simulink model "tanks"  (R2021b)
settings: Solver=ode45  StartTime=0.0  StopTime=200  RelTol=1e-6  EnableMultiTasking=on
values from neighbouring files (symbols this model uses):
  A_discretized = ssd.A    [control_design.m]
  B_discretized = ssd.B    [control_design.m]
  C = [0 , 1]    [control_design.m]
  C_discretized = ssd.C    [control_design.m]
  D_discretized = ssd.D    [control_design.m]
  F = tf(num, den)    [control_design.m]
  Gamma = sys_d.B    [control_design.m]
  K = acker(transpose(Phi), transpose(C), poles_desiredK).'    [control_design.m]
  L = acker(Phi, Gamma, poles_desiredL)    [control_design.m]
  lr = 1 / (C * inv(I - Phi + Gamma * L) * Gamma)    [control_design.m]
  Phi = sys_d.A    [control_design.m]
  Ts = 4    [control_design.m]
  uss = alpha2/beta*sqrt(2*g*tank_init_h2)*100/15    [control_design.m]
  yss = 40    [control_design.m]
undefined symbols (not defined in the file or in its folder): tank_A1, tank_a1, tank_A2, tank_a2, tank_H1, tank_H2, tank_init_h1, tank_init_h2, tank_Kpump
settings Model: Creator=lindhe  LastModifiedBy=1412
settings SolverCC: AlgebraicLoopSolver=TrustRegion
settings DataIOCC: LimitDataPoints=on  SaveFormat=Array  SignalLoggingSaveFormat=ModelDataLogs  ReturnWorkspaceOutputs=off  SignalLoggingName=sigsOut  Refine=3
settings OptimizationCC: ExpressionDepthLimit=2147483647  InitFltsAndDblsToZero=on  LifeSpan=inf
settings DebuggingCC: SaveWithParameterizedLinksMsg=none  UnderspecifiedInitializationDetection=Classic  MergeDetectMultiDrivingBlocksExec=none  SignalResolutionControl=TryResolveAllWithWarning  MultiTaskDSMMsg=warning  MultiTaskCondExecSysMsg=none  FcnCallInpInsideContextMsg=warning  StateNameClashWarn=warning  SFUnexpectedBacktrackingDiag=warning  SFNoUnconditionalDefaultTransitionDiag=warning  SFExecutionAtInitializationDiag=none  SFMachineParentedDataDiag=warning  ArithmeticOperatorsInVariantConditions=warning
settings HardwareCC: ProdBitPerPointer=32  ProdBitPerSizeT=32  ProdBitPerPtrDiffT=32  ProdLargestAtomicFloat=None  ProdIntDivRoundTo=Undefined  ProdEndianess=Unspecified  ProdWordSize=32  ProdHWDeviceType=32-bit Generic  TargetBitPerPointer=64  TargetBitPerSizeT=64  TargetBitPerPtrDiffT=64  TargetLongLongMode=on  TargetIntDivRoundTo=Zero  TargetEndianess=LittleEndian  TargetWordSize=64  TargetHWDeviceType=MATLAB Host  ProdEqTarget=off
settings ModelReferenceCC: PropagateSignalLabelsOutOfModel=off
settings SFSimCC: SimUseLocalCustomCode=off  CustomCodeUndefinedFunction=UseInterfaceOnly
settings RTWCC: SystemTargetFile=accel.tlc  TemplateMakefile=accel_default_tmf  RTWUseLocalCustomCode=off
settings CodeAppCC: StateflowObjectComments=on
settings STFCustomTargetCC: MATLABClassNameForMDSCustomization=Simulink.SoftwareTarget.TargetSpecificTriggerConfigurationBase  SystemTargetFile=accel.tlc
settings ConfigComp: CovMetricSettings=dw  CovSaveCumulativeToWorkspaceVar=on  CovSaveSingleToWorkspaceVar=on  CovExternalEMLEnable=off

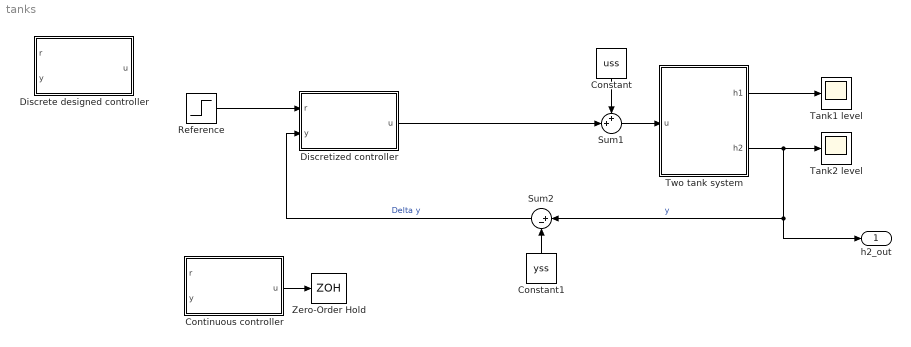
== system tanks ==
  Constant : Constant  Value=uss
  Constant1 : Constant  Value=yss
  Continuous controller : Subsystem
  Discrete designed controller : Subsystem
  Discretized controller : Subsystem
  Reference : Step  Time=25  After=10  SampleTime=0
  Sum1 : Sum  Inputs=++|
  Sum2 : Sum  Inputs=|+-
  Tank1 level : Scope
  Tank2 level : Scope
  Two tank system : Subsystem
  Zero-Order Hold : ZeroOrderHold  SampleTime=8
  h2_out : Outport
  wires:
  Constant/1 -> Sum1/1
  Two tank system/2(h2) -> Tank2 level/1, h2_out/1, Sum2/1  "y"
  Sum1/1 -> Two tank system/1(u)
  Two tank system/1(h1) -> Tank1 level/1
  Constant1/1 -> Sum2/2
  Sum2/1 -> Discretized controller/2(y)  "Delta y"
  Continuous controller/1(u) -> Zero-Order Hold/1
  Reference/1 -> Discretized controller/1(r)
  Discretized controller/1(u) -> Sum1/2

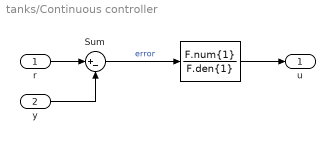
== system tanks/Continuous controller ==
  r : Inport
  y : Inport  Port=2
  " " : TransferFcn  Numerator=F.num{1}  Denominator=F.den{1}
  Sum : Sum  Inputs=|+-  SaturateOnIntegerOverflow=on
  u : Outport
  wires:
  Sum/1 -> " "/1  "error"
  y/1 -> Sum/2
  r/1 -> Sum/1
  " "/1 -> u/1

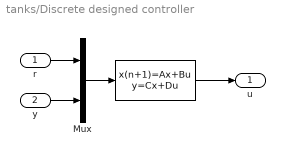
== system tanks/Discrete designed controller ==
  r : Inport
  y : Inport  Port=2
  " " : DiscreteStateSpace  A=Phi-Gamma*L-K*C  B=[lr * Gamma K]  C=-L  D=[lr 0]  SampleTime=Ts
  Mux : Mux  Inputs=2
  u : Outport
  wires:
  r/1 -> Mux/1
  y/1 -> Mux/2
  Mux/1 -> " "/1
  " "/1 -> u/1

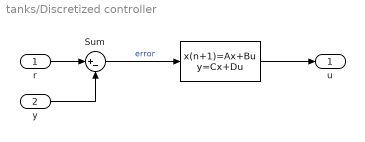
== system tanks/Discretized controller ==
  r : Inport
  y : Inport  Port=2
  " " : DiscreteStateSpace  A=A_discretized  B=B_discretized  C=C_discretized  D=D_discretized  SampleTime=Ts
  Sum : Sum  Inputs=|+-  SaturateOnIntegerOverflow=on
  u : Outport
  wires:
  Sum/1 -> " "/1  "error"
  y/1 -> Sum/2
  r/1 -> Sum/1
  " "/1 -> u/1

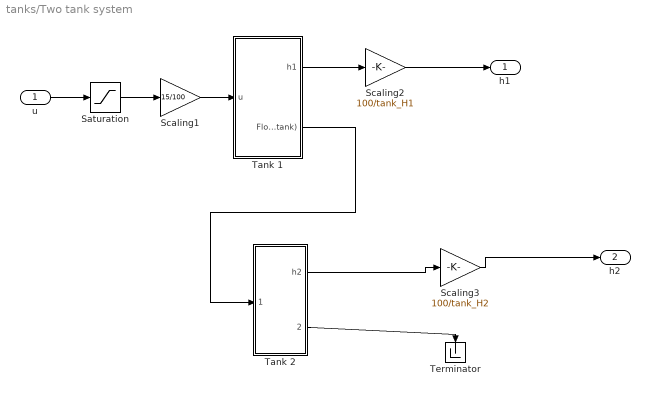
== system tanks/Two tank system ==
  u : Inport
  Saturation : Saturate  UpperLimit=100  LowerLimit=-0
  Scaling1 : Gain  Gain=15/100  SaturateOnIntegerOverflow=on  OutDataTypeStr=Inherit: Same as input  ParamDataTypeStr=Inherit: Same as input
  Scaling2 : Gain  Gain=100/tank_H1  SaturateOnIntegerOverflow=on  OutDataTypeStr=Inherit: Same as input  ParamDataTypeStr=Inherit: Same as input
  Scaling3 : Gain  Gain=100/tank_H2  SaturateOnIntegerOverflow=on  OutDataTypeStr=Inherit: Same as input  ParamDataTypeStr=Inherit: Same as input
  Tank 1 : Subsystem
  Tank 2 : Subsystem
  Terminator : Terminator
  h1 : Outport
  h2 : Outport  Port=2
  wires:
  Tank 2/1(h2) -> Scaling3/1
  Tank 2/2(Flow out) -> Terminator/1
  u/1 -> Saturation/1
  Tank 1/1(h1) -> Scaling2/1
  Tank 1/2(Flow out  (to lower tank)) -> Tank 2/1(From upper tank)
  Scaling2/1 -> h1/1
  Scaling3/1 -> h2/1
  Scaling1/1 -> Tank 1/1(u)
  Saturation/1 -> Scaling1/1

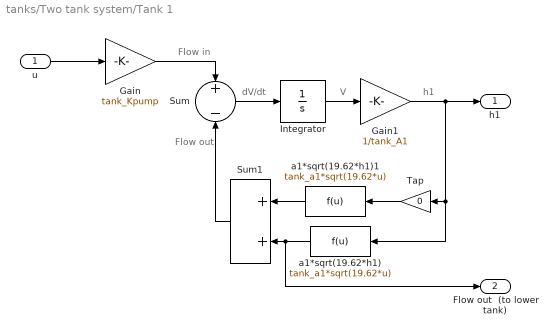
== system tanks/Two tank system/Tank 1 ==
  note: h1
  note: V
  note: dV/dt
  note: Flow out
  note: Flow in
  u : Inport
  Gain : Gain  Gain=tank_Kpump  SaturateOnIntegerOverflow=on  OutDataTypeStr=Inherit: Same as input  ParamDataTypeStr=Inherit: Same as input
  Gain1 : Gain  Gain=1/tank_A1  SaturateOnIntegerOverflow=on  OutDataTypeStr=Inherit: Same as input  ParamDataTypeStr=Inherit: Same as input
  Integrator : Integrator  InitialCondition=tank_init_h1*tank_A1  LimitOutput=on  UpperSaturationLimit=tank_H1*tank_A1  LowerSaturationLimit=0
  Sum : Sum  Inputs=+-  InputSameDT=on  SaturateOnIntegerOverflow=on  OutDataTypeStr=Inherit: Same as first input
  Sum1 : Sum  InputSameDT=on  SaturateOnIntegerOverflow=on  OutDataTypeStr=Inherit: Same as first input
  Tap : Gain  Gain=0  SaturateOnIntegerOverflow=on  OutDataTypeStr=Inherit: Same as input  ParamDataTypeStr=Inherit: Same as input
  a1*sqrt(19.62*h1) : Fcn  Expr=tank_a1*sqrt(19.62*u)
  a1*sqrt(19.62*h1)1 : Fcn  Expr=tank_a1*sqrt(19.62*u)
  h1 : Outport
  Flow out  (to lower tank) : Outport  Port=2
  wires:
  Gain1/1 -> Tap/1, a1*sqrt(19.62*h1)/1, h1/1
  Integrator/1 -> Gain1/1
  Sum/1 -> Integrator/1
  Gain/1 -> Sum/1
  u/1 -> Gain/1
  a1*sqrt(19.62*h1)/1 -> Flow out  (to lower tank)/1, Sum1/2
  a1*sqrt(19.62*h1)1/1 -> Sum1/1
  Sum1/1 -> Sum/2
  Tap/1 -> a1*sqrt(19.62*h1)1/1

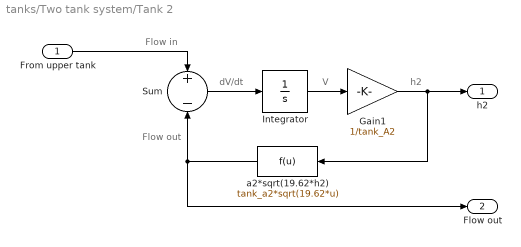
== system tanks/Two tank system/Tank 2 ==
  note: Flow in
  note: Flow out
  note: dV/dt
  note: V
  note: h2
  From upper tank : Inport
  Gain1 : Gain  Gain=1/tank_A2  SaturateOnIntegerOverflow=on  OutDataTypeStr=Inherit: Same as input  ParamDataTypeStr=Inherit: Same as input
  Integrator : Integrator  InitialCondition=tank_init_h2*tank_A2  LimitOutput=on  UpperSaturationLimit=tank_H2*tank_A2  LowerSaturationLimit=0
  Sum : Sum  Inputs=+-  InputSameDT=on  SaturateOnIntegerOverflow=on  OutDataTypeStr=Inherit: Same as first input
  a2*sqrt(19.62*h2) : Fcn  Expr=tank_a2*sqrt(19.62*u)
  h2 : Outport
  Flow out : Outport  Port=2
  wires:
  Sum/1 -> Integrator/1
  Integrator/1 -> Gain1/1
  Gain1/1 -> h2/1, a2*sqrt(19.62*h2)/1
  a2*sqrt(19.62*h2)/1 -> Sum/2, Flow out/1
  From upper tank/1 -> Sum/1
